simulink model "vel"  (R2020a)
settings: Solver=VariableStepAuto  StartTime=0  StopTime=600  RelTol=1e-3
values from neighbouring files (symbols this model uses):
  aeroDragCoeff = 0.38    [data.mat]
  airDensity = 1.23    [data.mat]
  frontArea = 2.1    [data.mat]
  gravity = 9.81    [data.mat]
  inclinationAngle = 0    [data.mat]
  intertialMassVeh = 2392    [data.mat]
  massVeh = 2300    [data.mat]
  rollingResistCoeff = 0.01    [data.mat]
undefined symbols (not defined in the file or in its folder): magnitude, modelG, Spinloss, wheelRadius
libraries: autolibshared x1, simulink x1
settings Model: Creator=khm  LastModifiedBy=khm

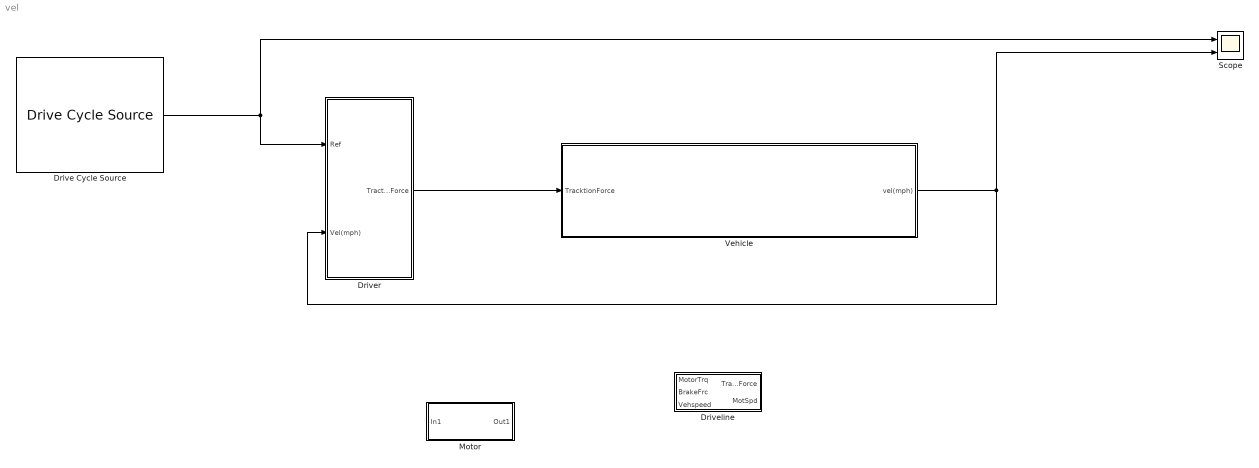
== system vel ==
  Drive Cycle Source : autolibshared/Drive Cycle Source  cycleVar=US06  fileVar=cycleFTP75.mat  tfinal="600  seconds"  cycleRepeat=off  outAccPort=off  outGearPort=off  gearList=No gear data  t_wot1=5  xdot_woto=0  xdot_wot1=30  t_wot2=20  xdot_wot2=0  t_wotend=30  srcUnit=m/s  outUnit=m/s  srcAccUnit=m/s/s  outAccUnit=m/s^2  dt=0  aMode=1  faultOption=off  velBnd=2  velBndUnit=mph  inUnit=m/s  timeBnd=1  failOption=off  stopSim=off  maxFaultCnt=10  maxFaultTime=2  maxTotFaultTime=15  traceOption=off  dtTrace=1  traceWindow=10  lastDCname=US06 Velocity  lastOutUnit=mph  lastDT=0  lastTB=1  lastSB=2  forceCalcBound=off
      settings: SourceProductBaseCode=PW,MT,VE,VP
  Driveline : Subsystem
  Driver : Subsystem
      mask Display: image("DriverPic.jpg")
  Motor : Subsystem
  Scope : Scope  NumInputPorts=2
  Vehicle : Subsystem
      mask Display: image("VehiclePic.jpg")
  wires:
  Drive Cycle Source/1 -> Scope/1, Driver/1(Ref)
  Driver/1(TractionForce) -> Vehicle/1(TracktionForce)
  Vehicle/1(vel(mph)) -> Scope/2, Driver/2(Vel(mph))

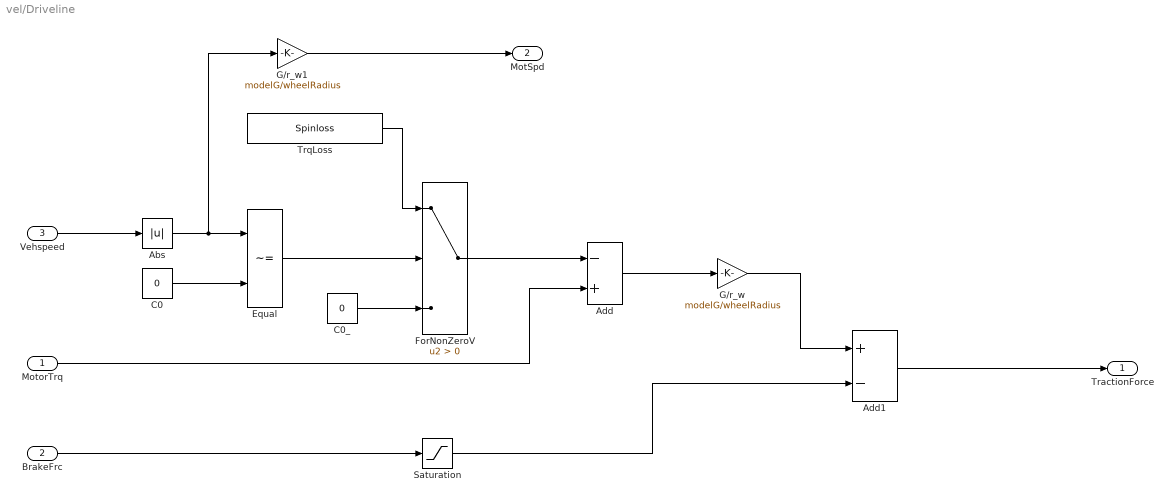
== system vel/Driveline ==
  MotorTrq : Inport
  BrakeFrc : Inport  Port=2
  Vehspeed : Inport  Port=3
  Abs : Abs
  Add : Sum  Inputs=-+
  Add1 : Sum  Inputs=+-
  C0 : Constant  Value=0
  C0_ : Constant  Value=0
  Equal : RelationalOperator  Operator=~=  OutDataTypeStr=boolean  RndMeth=Simplest
  ForNonZeroV : Switch  Criteria=u2 > Threshold
  G/r_w : Gain  Gain=modelG/wheelRadius
  G/r_w1 : Gain  Gain=modelG/wheelRadius
  Saturation : Saturate  UpperLimit=0  LowerLimit=-10000
  TrqLoss : Constant  Value=Spinloss
  TractionForce : Outport
  MotSpd : Outport  Port=2
  wires:
  Vehspeed/1 -> Abs/1
  Abs/1 -> G/r_w1/1, Equal/1
  C0/1 -> Equal/2
  Equal/1 -> ForNonZeroV/2
  TrqLoss/1 -> ForNonZeroV/1
  C0_/1 -> ForNonZeroV/3
  ForNonZeroV/1 -> Add/1
  MotorTrq/1 -> Add/2
  Add/1 -> G/r_w/1
  G/r_w/1 -> Add1/1
  BrakeFrc/1 -> Saturation/1
  Saturation/1 -> Add1/2
  Add1/1 -> TractionForce/1
  G/r_w1/1 -> MotSpd/1

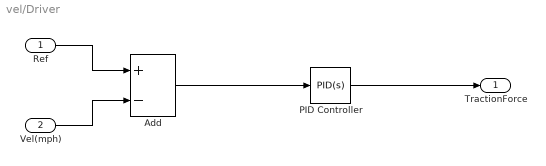
== system vel/Driver ==
  Ref : Inport
  Vel(mph) : Inport  Port=2
  Add : Sum  Inputs=+-
  PID Controller : simulink/Continuous/PID Controller  Controller=PID  Form=Parallel  TimeDomain=Continuous-time  UseExternalTs=off  SampleTime=-1  IntegratorMethod=Forward Euler  FilterMethod=Forward Euler  ControllerParametersSource=internal  P=7500  I=1  D=0  UseFilter=on  N=100  TunerSelectOption=Transfer Function Based (PID Tuner App)  InitialConditionSource=internal  InitialConditionForIntegrator=0  InitialConditionForFilter=0  DifferentiatorICPrevScaledInput=0  ExternalReset=none  TrackingMode=off  Kt=1  LimitOutput=off  UpperSaturationLimit=inf  LowerSaturationLimit=-inf  LinearizeAsGain=on  AntiWindupMode=none  Kb=1  POutMin=[]  POutMax=[]  IOutMin=[]  IOutMax=[]  DOutMin=[]  DOutMax=[]  NOutMin=[]  NOutMax=[]  SumOutMin=[]  SumOutMax=[]  SaturationOutMin=[]  SaturationOutMax=[]  PParamMin=[]  PParamMax=[]  IParamMin=[]  IParamMax=[]  DParamMin=[]  DParamMax=[]  NParamMin=[]  NParamMax=[]  KbParamMin=[]  KbParamMax=[]  KtParamMin=[]  KtParamMax=[]  KbOutMin=[]  KbOutMax=[]  KtOutMin=[]  KtOutMax=[]  IntegratorOutMin=[]  IntegratorOutMax=[]  FilterOutMin=[]  FilterOutMax=[]  SumI1OutMin=[]  SumI1OutMax=[]  SumI2OutMin=[]  SumI2OutMax=[]  SumI3OutMin=[]  SumI3OutMax=[]  SumI4OutMin=[]  SumI4OutMax=[]  SumDOutMin=[]  SumDOutMax=[]  DifferentiatorOutMin=[]  DifferentiatorOutMax=[]  FilterDiffOutCoefMin=[]  FilterDiffOutCoefMax=[]  ReciprocalOutMin=[]  ReciprocalOutMax=[]  SumDenOutMin=[]  SumDenOutMax=[]  SumNumOutMin=[]  SumNumOutMax=[]  DivideOutMin=[]  DivideOutMax=[]  UdiffTsProdOutMin=[]  UdiffTsProdOutMax=[]  NTsProdOutMin=[]  NTsProdOutMax=[]  UintegralTsProdOutMin=[]  UintegralTsProdOutMax=[]  UngainTsProdOutMin=[]  UngainTsProdOutMax=[]  IntegratorContinuousStateAttributes=''  IntegratorStateMustResolveToSignalObject=off  IntegratorRTWStateStorageClass=Auto  FilterContinuousStateAttributes=''  FilterStateMustResolveToSignalObject=off  FilterRTWStateStorageClass=Auto  ParallelPVariant=InternalParameters  IdealPVariant=Disabled  IVariant=InternalParameters  DVariant=InternalParameters  IntegratorVariant=Continuous  SatVariant=Disabled  AWVariant=Passthrough  PCopyVariant=Disabled  TRVariant=Disabled  FdbkBlocksVariant=Forward  IdealPFdbkVariant=Disabled  SatFdbkVariant=Disabled  DerivativeFilterVariant=ContFilter  NVariant=InternalParameters  NCopyVariant=Disabled  FilterICVariant=InternalICsFilter  IntegratorICVariant=InternalICs  ExternalResetVariant=Disabled  TRSumVariant=Passthrough  SumFdbkVariant=Disabled  SumVariant=Sum_PID  TsampFilterVariant=InternalTs  TsampNgainVariant=Passthrough  TsampIntegralVariant=Passthrough
  TractionForce : Outport
  wires:
  Ref/1 -> Add/1
  Vel(mph)/1 -> Add/2
  Add/1 -> PID Controller/1
  PID Controller/1 -> TractionForce/1

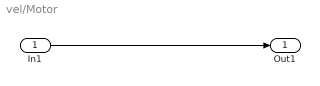
== system vel/Motor ==
  In1 : Inport
  Out1 : Outport
  wires:
  In1/1 -> Out1/1

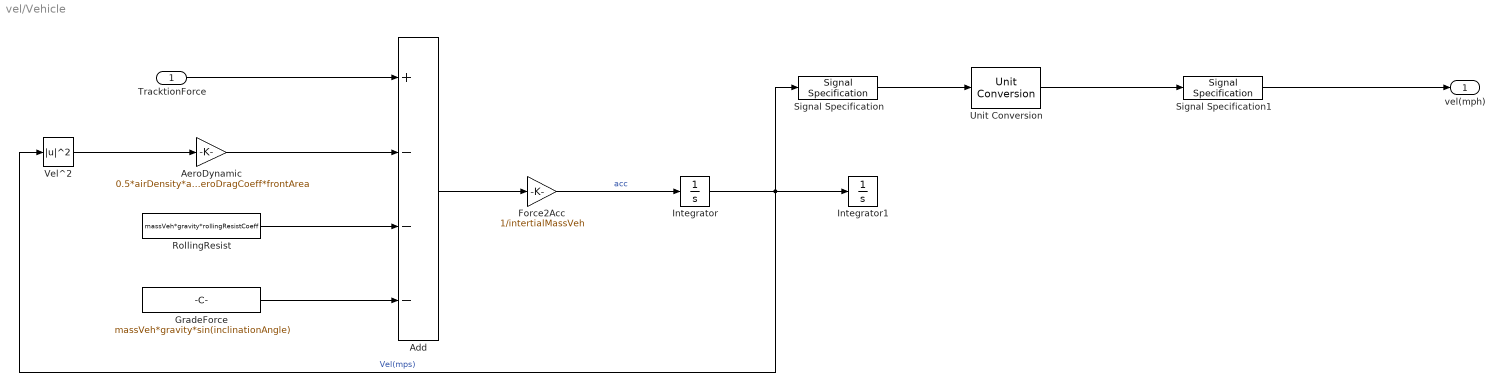
== system vel/Vehicle ==
  TracktionForce : Inport
  Add : Sum  Inputs=+---
  AeroDynamic : Gain  Gain=0.5*airDensity*aeroDragCoeff*frontArea
  Force2Acc : Gain  Gain=1/intertialMassVeh
  GradeForce : Constant  Value=massVeh*gravity*sin(inclinationAngle)
      settings: AttributesFormatString=%<Value>
  Integrator : Integrator
  Integrator1 : Integrator
  RollingResist : Constant  Value=massVeh*gravity*rollingResistCoeff
      settings: AttributesFormatString=%<Value>
  Signal Specification : SignalSpecification  Unit=m/s
  Signal Specification1 : SignalSpecification  Unit=m/h
  Unit Conversion : UnitConversion
  Vel^2 : Math  Operator=magnitude^2  SaturateOnIntegerOverflow=on
  vel(mph) : Outport
  wires:
  TracktionForce/1 -> Add/1
  GradeForce/1 -> Add/4
  RollingResist/1 -> Add/3
  AeroDynamic/1 -> Add/2
  Vel^2/1 -> AeroDynamic/1
  Add/1 -> Force2Acc/1
  Force2Acc/1 -> Integrator/1  "acc"
  Integrator/1 -> Signal Specification/1, Vel^2/1, Integrator1/1  "Vel(mps)"
  Signal Specification/1 -> Unit Conversion/1
  Unit Conversion/1 -> Signal Specification1/1
  Signal Specification1/1 -> vel(mph)/1
